simulink model "kadai13"  (R2021b)
settings: Solver=VariableStepAuto  StartTime=0.0  StopTime=10.0  MaxStep=0.01  RelTol=1e-10
settings Model: Creator=is221042  LastModifiedBy=tomotomo

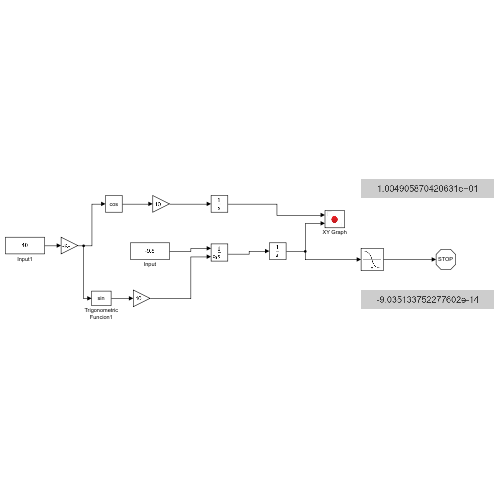
[thumbnail: Simulink's stored preview of the top-level diagram]
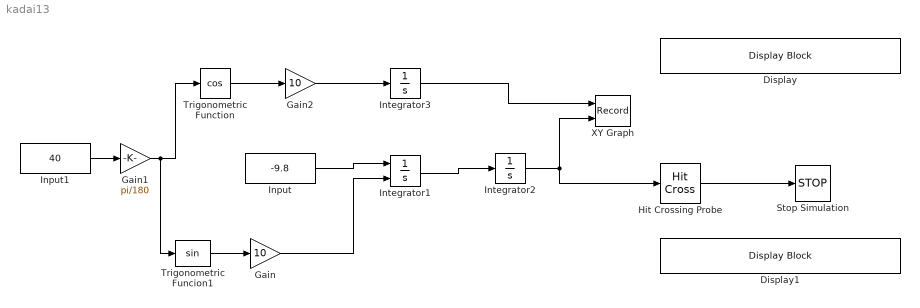
== system kadai13 ==
  Display : DisplayBlock  LabelPosition=Hide  Format=longE  Transparency=1
  Display1 : DisplayBlock  LabelPosition=Hide  Format=longE  Transparency=1
  Gain : Gain  Gain=10
  Gain1 : Gain  Gain=pi/180
  Gain2 : Gain  Gain=10
  Hit Crossing Probe : HitCross  HitCrossingDirection=falling
  Input : Constant  Value=-9.8
  Input1 : Constant  Value=40
  Integrator1 : Integrator  InitialConditionSource=external  InitialCondition=12
  Integrator2 : Integrator
  Integrator3 : Integrator
  Stop Simulation : Stop
  Trigonometric Funcion1 : Trigonometry
  Trigonometric Function : Trigonometry  Operator=cos
  XY Graph : Record  FileSettingsInternal="{\"entries\":[{\"content\":{\"excelSettings\":{\"content\":{},\"type\":\"Streamout.ExcelSettings\"}},\"type\":\"Streamout.FileSettingStorage\",\"uuid\":\"76204225-9850-494e-8b36-159b5771198a\"}],\"packageUris\":[\"http://schema.mathworks.com/mf0/streamout_blocks/R2020a\"],\"version\":\"1.0\"}"  Layout=[1 1]  SignalsInternal="{\"entries\":[{\"content\":{\"signals\":[{\"content\":{\"blockPath\":[\"kadai13/XY Graph\"],\"channel\":[],\"dimensions\":[1],\"domain\":\"kadai13/XY Graph\",\"lineColor\":\"#a2142f\",\"plots\":[1],\"port\":1,\"sid\":[\"\"],\"signalID\":529,\"signalName\":\"Integrator3\"},\"type\":\"RecordBlkView.Signal\",\"uuid\":\"fd7c2e25-95cd-4684-b1da-ebae4ffeb50d\"},{\"content\":{\"blockPath\":[\"kadai13/XY Graph\"],\"channel\":[],\"dimensions\":[1],\"domain\":\"kadai13/XY Graph\",\"lineColor\":\"#139fff\",\"plots\":[1],\"port\":2,\"sid\":[\"\"],\"signalID\":533,\"signalName\":\"Integrator2\"},\"type\":\"RecordBlkView.Signal\",\"uuid\":\"21d1692d-99e8-4bf1-b75c-240c9dde113c\"}]},\"type\":\"RecordBlkView.InputSignals\",\"uuid\":\"008c63c1-7923-46d5-b493-328521c03786\"}],\"packageUris\":[\"http://schema.mathworks.com/mf0/streamout_blocks/R2020a\"],\"version\":\"1.0\"}"  VisualizationBindings="{\"xyplotplugin\":{\"info\":[{\"series\":[{\"bindingParametersList\":[{\"parameter\":\"X-Axis\",\"signalID\":529,\"signalName\":\"Integrator3\"},{\"parameter\":\"Y-Axis\",\"signalID\":533,\"signalName\":\"Integrator2\"}],\"seriesID\":32138}],\"subplotID\":1}]}}"  CompatibilityTag=XY
  wires:
  Integrator1/1 -> Integrator2/1
  Hit Crossing Probe/1 -> Stop Simulation/1
  Integrator2/1 -> XY Graph/2, Hit Crossing Probe/1
  Input/1 -> Integrator1/1
  Integrator3/1 -> XY Graph/1
  Trigonometric Function/1 -> Gain2/1
  Gain/1 -> Integrator1/2
  Input1/1 -> Gain1/1
  Gain2/1 -> Integrator3/1
  Trigonometric Funcion1/1 -> Gain/1
  Gain1/1 -> Trigonometric Funcion1/1, Trigonometric Function/1
